simulink library "ESD_CAN_lib"  (Simulink 7.1)
libraries: xpclib x5
settings Model: Creator=ilMaggia  LastModifiedBy=ilMaggia

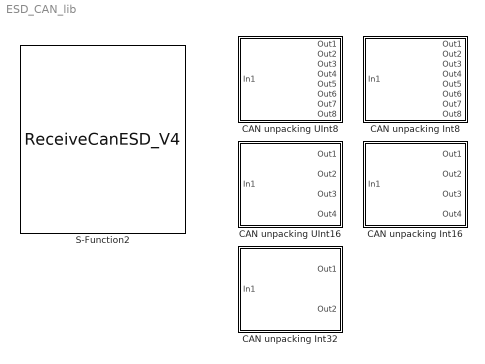
== system ESD_CAN_lib ==
  CAN unpacking Int16 : Subsystem
  CAN unpacking Int32 : Subsystem
  CAN unpacking Int8 : Subsystem
  CAN unpacking UInt16 : Subsystem
  CAN unpacking UInt8 : Subsystem
  S-Function2 : S-Function  FunctionName=ReceiveCanESD_V4  Parameters=(baudrate),msgID  EnableBusSupport=off  mask{msgID=[768:770], baudrate=1000 Kbits/s}
      mask prompts: msgID "Message ID"
      mask StyleString: edit,popup(1000 Kbits/s|800  Kbits/s|666.6Kbits/s|500  Kbits/s)
      mask Display:
      | fprintf('RECEIVE CAN\n\n\n')
      | fprintf('\nID %d',msgID);

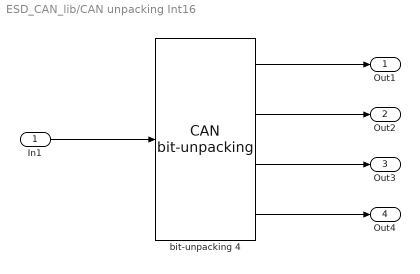
== system ESD_CAN_lib/CAN unpacking Int16 ==
  In1 : Inport  OutDataType=sfix(16)  OutScaling=2^0
  " bit-unpacking 4" : xpclib/CAN/Utilities/CAN bit-unpacking   bitpatterns={[0:15] [16:31] [32:47] [48:63]}  dtypes="{'Int16' 'Int16' 'Int16'  'Int16'}"
  Out1 : Outport  OutDataType=sfix(16)  OutScaling=2^0
  Out2 : Outport  Port=2  OutDataType=sfix(16)  OutScaling=2^0
  Out3 : Outport  Port=3  OutDataType=sfix(16)  OutScaling=2^0
  Out4 : Outport  Port=4  OutDataType=sfix(16)  OutScaling=2^0
  wires:
  " bit-unpacking 4"/4 -> Out4/1
  " bit-unpacking 4"/3 -> Out3/1
  " bit-unpacking 4"/2 -> Out2/1
  " bit-unpacking 4"/1 -> Out1/1
  In1/1 -> " bit-unpacking 4"/1

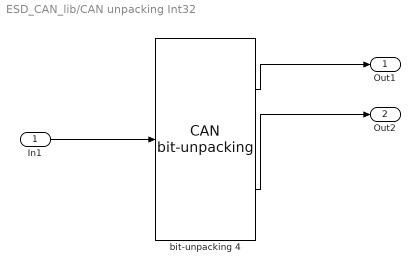
== system ESD_CAN_lib/CAN unpacking Int32 ==
  In1 : Inport  OutDataType=sfix(16)  OutScaling=2^0
  " bit-unpacking 4" : xpclib/CAN/Utilities/CAN bit-unpacking   bitpatterns={[0:31] [32:63]}  dtypes={'int32' 'int32' }
  Out1 : Outport  OutDataType=sfix(16)  OutScaling=2^0
  Out2 : Outport  Port=2  OutDataType=sfix(16)  OutScaling=2^0
  wires:
  " bit-unpacking 4"/2 -> Out2/1
  " bit-unpacking 4"/1 -> Out1/1
  In1/1 -> " bit-unpacking 4"/1

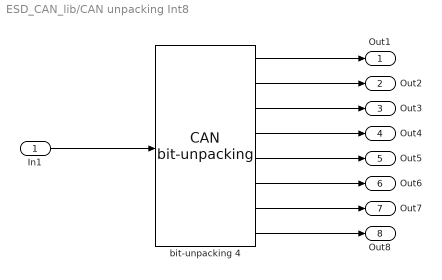
== system ESD_CAN_lib/CAN unpacking Int8 ==
  In1 : Inport  OutDataType=sfix(16)  OutScaling=2^0
  " bit-unpacking 4" : xpclib/CAN/Utilities/CAN bit-unpacking   bitpatterns={[0:7] [8:15] [16:23] [24:31] [32:39] [40:47] [48:55] [56:63]}  dtypes="{'int8' 'int8' 'int8'  'int8' 'int8' 'int8' 'int8' 'int8'}"
  Out1 : Outport  OutDataType=sfix(16)  OutScaling=2^0
  Out2 : Outport  Port=2  OutDataType=sfix(16)  OutScaling=2^0
  Out3 : Outport  Port=3  OutDataType=sfix(16)  OutScaling=2^0
  Out4 : Outport  Port=4  OutDataType=sfix(16)  OutScaling=2^0
  Out5 : Outport  Port=5  OutDataType=sfix(16)  OutScaling=2^0
  Out6 : Outport  Port=6  OutDataType=sfix(16)  OutScaling=2^0
  Out7 : Outport  Port=7  OutDataType=sfix(16)  OutScaling=2^0
  Out8 : Outport  Port=8  OutDataType=sfix(16)  OutScaling=2^0
  wires:
  In1/1 -> " bit-unpacking 4"/1
  " bit-unpacking 4"/1 -> Out1/1
  " bit-unpacking 4"/2 -> Out2/1
  " bit-unpacking 4"/3 -> Out3/1
  " bit-unpacking 4"/4 -> Out4/1
  " bit-unpacking 4"/5 -> Out5/1
  " bit-unpacking 4"/6 -> Out6/1
  " bit-unpacking 4"/7 -> Out7/1
  " bit-unpacking 4"/8 -> Out8/1

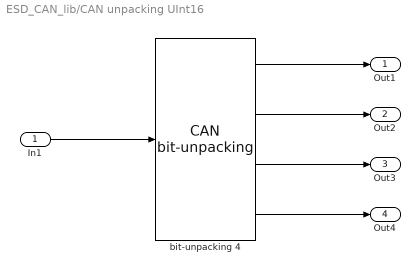
== system ESD_CAN_lib/CAN unpacking UInt16 ==
  In1 : Inport  OutDataType=sfix(16)  OutScaling=2^0
  " bit-unpacking 4" : xpclib/CAN/Utilities/CAN bit-unpacking   bitpatterns={[0:15] [16:31] [32:47] [48:63]}  dtypes="{'uint16' 'uint16' 'uint16'  'uint16'}"
  Out1 : Outport  OutDataType=sfix(16)  OutScaling=2^0
  Out2 : Outport  Port=2  OutDataType=sfix(16)  OutScaling=2^0
  Out3 : Outport  Port=3  OutDataType=sfix(16)  OutScaling=2^0
  Out4 : Outport  Port=4  OutDataType=sfix(16)  OutScaling=2^0
  wires:
  In1/1 -> " bit-unpacking 4"/1
  " bit-unpacking 4"/1 -> Out1/1
  " bit-unpacking 4"/2 -> Out2/1
  " bit-unpacking 4"/3 -> Out3/1
  " bit-unpacking 4"/4 -> Out4/1

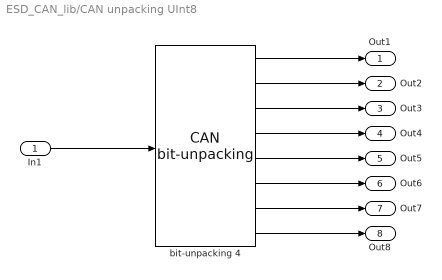
== system ESD_CAN_lib/CAN unpacking UInt8 ==
  In1 : Inport  OutDataType=sfix(16)  OutScaling=2^0
  " bit-unpacking 4" : xpclib/CAN/Utilities/CAN bit-unpacking   bitpatterns={[0:7] [8:15] [16:23] [24:31] [32:39] [40:47] [48:55] [56:63]}  dtypes="{'uint8' 'uint8' 'uint8'  'uint8' 'uint8' 'uint8' 'uint8' 'uint8'}"
  Out1 : Outport  OutDataType=sfix(16)  OutScaling=2^0
  Out2 : Outport  Port=2  OutDataType=sfix(16)  OutScaling=2^0
  Out3 : Outport  Port=3  OutDataType=sfix(16)  OutScaling=2^0
  Out4 : Outport  Port=4  OutDataType=sfix(16)  OutScaling=2^0
  Out5 : Outport  Port=5  OutDataType=sfix(16)  OutScaling=2^0
  Out6 : Outport  Port=6  OutDataType=sfix(16)  OutScaling=2^0
  Out7 : Outport  Port=7  OutDataType=sfix(16)  OutScaling=2^0
  Out8 : Outport  Port=8  OutDataType=sfix(16)  OutScaling=2^0
  wires:
  " bit-unpacking 4"/8 -> Out8/1
  " bit-unpacking 4"/7 -> Out7/1
  " bit-unpacking 4"/6 -> Out6/1
  " bit-unpacking 4"/5 -> Out5/1
  " bit-unpacking 4"/4 -> Out4/1
  " bit-unpacking 4"/3 -> Out3/1
  " bit-unpacking 4"/2 -> Out2/1
  " bit-unpacking 4"/1 -> Out1/1
  In1/1 -> " bit-unpacking 4"/1
